simulink model "frequenzbereich"  (R2020a)
settings: Solver=ode23s  StartTime=0.0  StopTime=20  RelTol=1e-3
undefined symbols (not defined in the file or in its folder): G_den, G_num, K_x_den, K_x_num
libraries: cstblocks x2
settings Model: Creator=niko  LastModifiedBy=niko

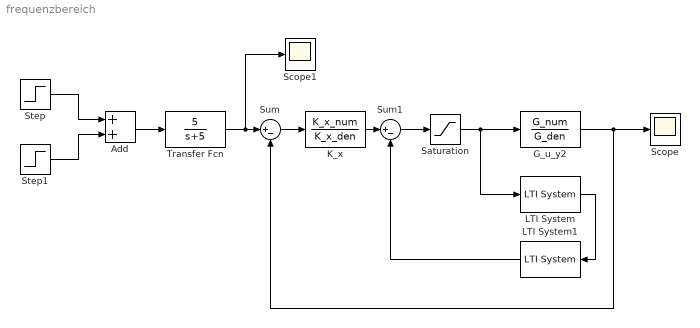
== system frequenzbereich ==
  Add : Sum
  G_u_y2 : TransferFcn  Numerator=G_num  Denominator=G_den
  K_x : TransferFcn  Numerator=K_x_num  Denominator=K_x_den
  LTI System : cstblocks/LTI System  sys=K_phi  IC=[]
  LTI System1 : cstblocks/LTI System  sys=G_u_y1  IC=[]
  Saturation : Saturate  UpperLimit=0.4  LowerLimit=-0.4
  Scope : Scope
  Scope1 : Scope
  Step : Step  SampleTime=0
  Step1 : Step  Time=10  After=-5  SampleTime=0
  Sum : Sum  Inputs=|+-
  Sum1 : Sum  Inputs=|+-
  Transfer Fcn : TransferFcn  Numerator=[5]  Denominator=[1 5]
  wires:
  G_u_y2/1 -> Scope/1, Sum/2
  Step/1 -> Add/1
  Step1/1 -> Add/2
  Sum/1 -> K_x/1
  Add/1 -> Transfer Fcn/1
  K_x/1 -> Sum1/1
  Sum1/1 -> Saturation/1
  LTI System1/1 -> Sum1/2
  LTI System/1 -> LTI System1/1
  Transfer Fcn/1 -> Scope1/1, Sum/1
  Saturation/1 -> LTI System/1, G_u_y2/1
